simulink model "controller_class"  (R2024a)
settings: Solver=ode45  StartTime=0.0  StopTime=10  RelTol=1e-3
undefined symbols (not defined in the file or in its folder): Bi, BL, Bm_r, Bo, cmd, dis, f_t, J_r, Ji, Jo, K1_B, K1_B_H2, K2_B, K2_B_H2, K_A, K_A_H2, K_C, K_C_H2, KD_H2, Kd_w, Ke_r, Ki_d, KI_H2, Ki_i, Ki_w, KJB, KP_H2, Kp_i, Kp_w, Ks, Kt_r, L_r, R0, R_r, Ri, Ro, t_t, Vdc, Vp
libraries: simulink x2, fuzblock x1
settings Model: Creator=yanqi  LastModifiedBy=yanqi

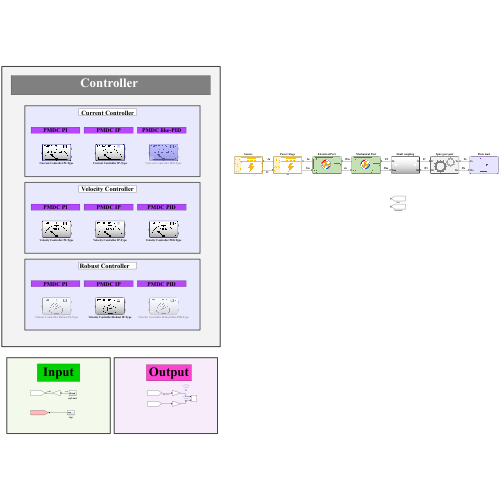
[thumbnail: Simulink's stored preview of the top-level diagram]
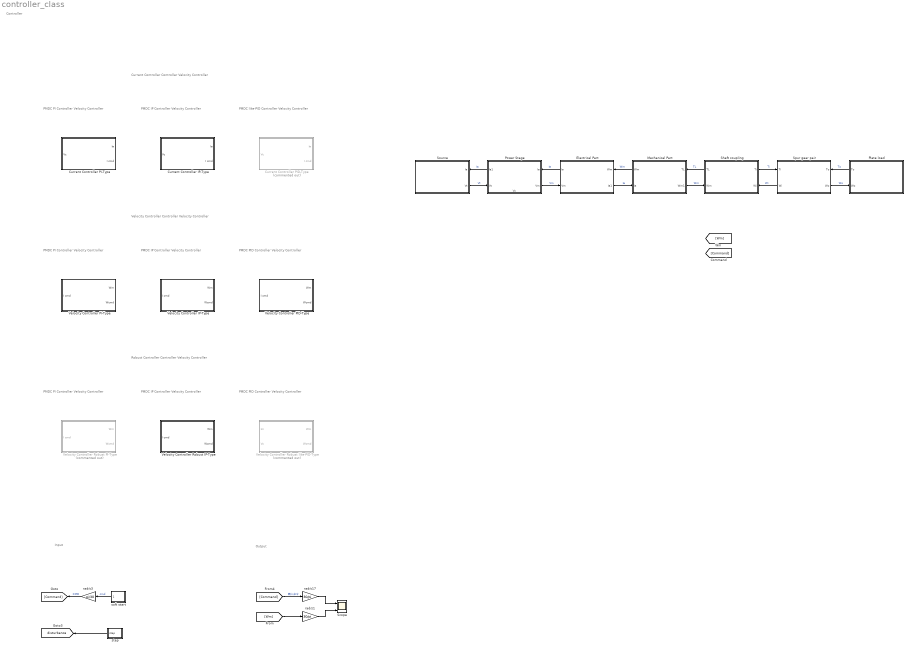
== system controller_class ==
  note: Current Controller Controller Velocity Controller
  note: PMDC IP Controller Velocity Controller
  note: PMDC like-PID Controller Velocity Controller
  note: PMDC PI Controller Velocity Controller
  note: Velocity Controller Controller Velocity Controller
  note: PMDC IP Controller Velocity Controller
  note: PMDC PID Controller Velocity Controller
  note: PMDC PI Controller Velocity Controller
  note: Robust Controller Controller Velocity Controller
  note: PMDC IP Controller Velocity Controller
  note: PMDC PID Controller Velocity Controller
  note: PMDC PI Controller Velocity Controller
  note: Controller
  note: Output
  note: Input
  Current Controller IP-Type : Subsystem  InitFcn=""
      mask Display: image("C:\Users\yanqi\Dropbox\強健控制\強健控制器設計\強健控制程式工具\TWO Port 模擬檔\可視化圖片\控制器\PMDC_Current_IP.png");
  Current Controller PI-Type : Subsystem  InitFcn=""
      mask Display: image("C:\Users\yanqi\Dropbox\強健控制\強健控制器設計\強健控制程式工具\TWO Port 模擬檔\可視化圖片\控制器\PMDC_Current_PI.png");
  Current Controller PID-Type : Subsystem  Commented=on  InitFcn=""
      mask Display: image("C:\Users\yanqi\Dropbox\強健控制\強健控制器設計\強健控制程式工具\TWO Port 模擬檔\可視化圖片\控制器\PMDC_Current_PID.png");
  Electrical Part : Subsystem
      settings: PortSchema="{\"entries\":[{\"content\":{\"sides\":[{\"content\":{\"connectorIds\":[\"Out2\",\"In1\"]},\"type\":\"ConnectorPlacement.EquallySpacedRectSide\",\"uuid\":\"f8a1ffa4-7450-4f3a-a88f-322599fa6d56\"},{\"content\":{\"connectorIds\":[\"In2\",\"Out1\"],\"side\":\"RIGHT\"},\"type\":\"ConnectorPlacement.EquallySpacedRectSide\",\"uuid\":\"f89fbec4-8dee-4bae-8289-3af4287f7f86\"},{\"content\":{\"side\":\"TOP\"},\"type\":\"ConnectorPlacement.EquallySpacedRectSide\",\"uuid\":\"83195871-21ad-4509-9495-08e0be9a8292\"}]},\"type\":\"ConnectorPlacement.EquallySpacedConnector\",\"uuid\":\"f8e5f4c3-4a70-47c9-aad6-1e160c7a2ed2\"}],\"packageUris\":[\"http://schema.mathworks.com/mf0/Connector/R2020b\"],\"version\":\"1.0\"}"
      mask Display: image('PMDC.png');
  Mechanical Part : Subsystem
      settings: PortSchema="{\"entries\":[{\"content\":{\"sides\":[{\"content\":{\"connectorIds\":[\"Out2\",\"In1\"]},\"type\":\"ConnectorPlacement.EquallySpacedRectSide\",\"uuid\":\"f8a1ffa4-7450-4f3a-a88f-322599fa6d56\"},{\"content\":{\"connectorIds\":[\"In2\",\"Out1\"],\"side\":\"RIGHT\"},\"type\":\"ConnectorPlacement.EquallySpacedRectSide\",\"uuid\":\"f89fbec4-8dee-4bae-8289-3af4287f7f86\"},{\"content\":{\"side\":\"TOP\"},\"type\":\"ConnectorPlacement.EquallySpacedRectSide\",\"uuid\":\"83195871-21ad-4509-9495-08e0be9a8292\"}]},\"type\":\"ConnectorPlacement.EquallySpacedConnector\",\"uuid\":\"f8e5f4c3-4a70-47c9-aad6-1e160c7a2ed2\"}],\"packageUris\":[\"http://schema.mathworks.com/mf0/Connector/R2020b\"],\"version\":\"1.0\"}"
      mask Display: image('PMDC.png');
  Plate load : Subsystem
      settings: PortSchema="{\"entries\":[{\"content\":{\"sides\":[{\"content\":{},\"type\":\"ConnectorPlacement.EquallySpacedRectSide\",\"uuid\":\"d42fc156-06c9-4c30-b734-ba7c649bcd6c\"},{\"content\":{\"side\":\"RIGHT\"},\"type\":\"ConnectorPlacement.EquallySpacedRectSide\",\"uuid\":\"e3421591-54ab-4525-97e2-f729a89143d8\"},{\"content\":{\"connectorIds\":[\"Out1\",\"In1\"],\"side\":\"TOP\"},\"type\":\"ConnectorPlacement.EquallySpacedRectSide\",\"uuid\":\"958f7cdf-8dcf-4bff-be32-b737eb42e197\"}]},\"type\":\"ConnectorPlacement.EquallySpacedConnector\",\"uuid\":\"ee7151ba-f83a-4c95-85b6-9993354922b3\"}],\"packageUris\":[\"http://schema.mathworks.com/mf0/Connector/R2020b\"],\"version\":\"1.0\"}"
      mask Display: image('LOAD.png');
  Power Stage : Subsystem
      settings: PortSchema="{\"entries\":[{\"content\":{\"sides\":[{\"content\":{\"connectorIds\":[\"Out2\",\"In1\"]},\"type\":\"ConnectorPlacement.EquallySpacedRectSide\",\"uuid\":\"58508ce2-1894-42d8-835a-89d3025a2a64\"},{\"content\":{\"connectorIds\":[\"In3\",\"Out1\"],\"side\":\"RIGHT\"},\"type\":\"ConnectorPlacement.EquallySpacedRectSide\",\"uuid\":\"6994be33-a1a7-4027-bab1-df4ce47b873a\"},{\"content\":{\"side\":\"TOP\"},\"type\":\"ConnectorPlacement.EquallySpacedRectSide\",\"uuid\":\"2ad4f745-7ac4-4e1a-9a98-a432c01e08ff\"},{\"content\":{\"connectorIds\":[\"In2\"],\"side\":\"BOTTOM\"},\"type\":\"ConnectorPlacement.EquallySpacedRectSide\",\"uuid\":\"1b30d730-4089-4eab-8923-76d29eb9f10c\"}]},\"type\":\"ConnectorPlacement.EquallySpacedConnector\",\"uuid\":\"b52e3181-20dc-4fdc-95a1-9a3597bd758e\"}],\"packageUris\":[\"http://schema.mathworks.com/mf0/Connector/R2020b\"],\"version\":\"1.0\"}"
      mask Display: image('DC Power.png');
  Scope : Scope  NumInputPorts=2
  Shaft coupling : Subsystem
      settings: PortSchema="{\"entries\":[{\"content\":{\"sides\":[{\"content\":{\"connectorIds\":[\"Out2\",\"In1\"]},\"type\":\"ConnectorPlacement.EquallySpacedRectSide\",\"uuid\":\"01ede124-f7d4-4ffa-a713-cf07b9ad0f27\"},{\"content\":{\"connectorIds\":[\"Out1\",\"In2\"],\"side\":\"RIGHT\"},\"type\":\"ConnectorPlacement.EquallySpacedRectSide\",\"uuid\":\"f66caf2a-ca8f-4ebf-97ad-d73b5315af29\"},{\"content\":{\"side\":\"TOP\"},\"type\":\"ConnectorPlacement.EquallySpacedRectSide\",\"uuid\":\"58e7144f-6e7e-4352-98b7-aac542d17719\"}]},\"type\":\"ConnectorPlacement.EquallySpacedConnector\",\"uuid\":\"1e1b0c9a-4571-49a4-a41d-a8591e57bca4\"}],\"packageUris\":[\"http://schema.mathworks.com/mf0/Connector/R2020b\"],\"version\":\"1.0\"}"
      mask Display: image('Rigid Coupling.png');
  Source : Subsystem
      settings: PortSchema="{\"entries\":[{\"content\":{\"sides\":[{\"content\":{},\"type\":\"ConnectorPlacement.EquallySpacedRectSide\",\"uuid\":\"717e91a0-288b-4ba5-84da-f262c24688bc\"},{\"content\":{\"connectorIds\":[\"In1\",\"Out1\"],\"side\":\"RIGHT\"},\"type\":\"ConnectorPlacement.EquallySpacedRectSide\",\"uuid\":\"569ee505-38fb-400b-9e45-0fafedafb0f3\"},{\"content\":{\"side\":\"TOP\"},\"type\":\"ConnectorPlacement.EquallySpacedRectSide\",\"uuid\":\"44407c3d-239d-4fc9-b2d2-10ddbad2f525\"}]},\"type\":\"ConnectorPlacement.EquallySpacedConnector\",\"uuid\":\"e894aa65-7991-48d5-91da-50bab94327d3\"}],\"packageUris\":[\"http://schema.mathworks.com/mf0/Connector/R2020b\"],\"version\":\"1.0\"}"
      mask Display: image('DC Power.png');
  Spur gear pair : Subsystem
      settings: PortSchema="{\"entries\":[{\"content\":{\"sides\":[{\"content\":{\"connectorIds\":[\"In1\",\"Out2\"]},\"type\":\"ConnectorPlacement.EquallySpacedRectSide\",\"uuid\":\"9ad50964-c829-49ed-8028-dcb862de1bdd\"},{\"content\":{\"connectorIds\":[\"In2\",\"Out1\"],\"side\":\"RIGHT\"},\"type\":\"ConnectorPlacement.EquallySpacedRectSide\",\"uuid\":\"a1a8b250-47a3-4252-871c-028bd872c8ce\"},{\"content\":{\"side\":\"TOP\"},\"type\":\"ConnectorPlacement.EquallySpacedRectSide\",\"uuid\":\"bcffd697-c189-4993-a911-6095dd8b92d6\"}]},\"type\":\"ConnectorPlacement.EquallySpacedConnector\",\"uuid\":\"be779869-a0ea-4cde-9a54-80cee426721f\"}],\"packageUris\":[\"http://schema.mathworks.com/mf0/Connector/R2020b\"],\"version\":\"1.0\"}"
      mask Display: image('Gear.png');
  Velocity Controller IP-Type : Subsystem  InitFcn=""
      mask Display: image("C:\Users\yanqi\Dropbox\強健控制\強健控制器設計\強健控制程式工具\TWO Port 模擬檔\可視化圖片\控制器\PMDC_Spped_IP.png");
  Velocity Controller PI-Type : Subsystem  InitFcn=""
      mask Display: image("C:\Users\yanqi\Dropbox\強健控制\強健控制器設計\強健控制程式工具\TWO Port 模擬檔\可視化圖片\控制器\PMDC_Spped_PI.png");
  Velocity Controller PID-Type : Subsystem  InitFcn=""
      mask Display: image("C:\Users\yanqi\Dropbox\強健控制\強健控制器設計\強健控制程式工具\TWO Port 模擬檔\可視化圖片\控制器\PMDC_Spped_PID.png");
  Velocity Controller Robust IP-Type : Subsystem  InitFcn=""
      mask Display: image("C:\Users\yanqi\Dropbox\強健控制\強健控制器設計\強健控制程式工具\TWO Port 模擬檔\可視化圖片\控制器\PMDC_Robust_IP.png");
  Velocity Controller Robust PI-Type : Subsystem  Commented=on  InitFcn=|
      | % P Matrix
      | H2_P = [-0.0953	0	0	1.9459	363.9515
      |         -1.0000	0	0.3410	-0.0021	0
      |         0	999.9800	0	0	0
      |         -0.2155	0	0	0	0
      |         0	0	0	0	0.0026
      |         0	1.0000	0.0011	0	0
      |         1.0000	0	0	0.0021	0];
      | 
      | %% H2 tool
      | [H2_A_T,H2_B_T,H2_C_T,H2_D_T,H2_A_K,H2_B_K,H2_C_K,H2_D_K,Norm] = H2_DF(H2_P,2,2,1,3,2);
      | 
      | % velocity controller
      | K_A_H2  = H2_A_K;
      | K1_B_H2 = H2_B_K(1:2,1);
      | K2_B_H2 = H2_B_K(1:2,2);
      | K_C_H2  = H2_C_K;
      mask Display: image("C:\Users\yanqi\Dropbox\強健控制\強健控制器設計\強健控制程式工具\TWO Port 模擬檔\可視化圖片\控制器\PMDC_Robust_PI.png");
  Velocity Controller Robust like-PID-Type : Subsystem  Commented=on  InitFcn=|
      | % P Matrix
      | H2_P = [-0.0953	0	0	1.9459	363.9515
      |         -1.0000	0	0.3410	-0.0021	0
      |         0	999.9800	0	0	0
      |         -0.2155	0	0	0	0
      |         0	0	0	0	0.0026
      |         0	1.0000	0.0011	0	0
      |         1.0000	0	0	0.0021	0];
      | 
      | %% H2 tool
      | [H2_A_T,H2_B_T,H2_C_T,H2_D_T,H2_A_K,H2_B_K,H2_C_K,H2_D_K,Norm] = H2_DF(H2_P,2,2,1,3,2);
      | 
      | % velocity controller
      | K_A_H2  = H2_A_K;
      | K1_B_H2 = H2_B_K(1:2,1);
      | K2_B_H2 = H2_B_K(1:2,2);
      | K_C_H2  = H2_C_K;
      settings: PortSchema="{\"entries\":[{\"content\":{\"sides\":[{\"content\":{\"connectorIds\":[\"In1\",\"In2\"]},\"type\":\"ConnectorPlacement.EquallySpacedRectSide\",\"uuid\":\"67442645-cd32-4145-b143-2bfd4b8863c1\"},{\"content\":{\"connectorIds\":[\"In3\",\"Out1\"],\"side\":\"RIGHT\"},\"type\":\"ConnectorPlacement.EquallySpacedRectSide\",\"uuid\":\"525717ef-81e8-4055-8109-230bda9ce61c\"},{\"content\":{\"side\":\"TOP\"},\"type\":\"ConnectorPlacement.EquallySpacedRectSide\",\"uuid\":\"18f89565-0718-45fc-8263-cc7fc51687c0\"}]},\"type\":\"ConnectorPlacement.EquallySpacedConnector\",\"uuid\":\"5a159387-e0fa-4e2f-b611-20c995e77047\"}],\"packageUris\":[\"http://schema.mathworks.com/mf0/Connector/R2020b\"],\"version\":\"1.0\"}"
      mask Display: image("C:\Users\yanqi\Dropbox\強健控制\強健控制器設計\強健控制程式工具\TWO Port 模擬檔\可視化圖片\控制器\PMDC_Robust_like-PID.png");
  rad/s1 : Gain  Gain=30/pi
  rad/s17 : Gain  Gain=30/pi
  rad/s3 : Gain  Gain=pi/30
  soft start : Subsystem
  step : Subsystem
  tag scope: disturbance=global
  wires:
  Shaft coupling/2(TL) -> Mechanical Part/2(TL)  "TL"
  Mechanical Part/1(Wm1) -> Shaft coupling/1(Wm)  "Wm"
  Source/1(Vt) -> Power Stage/1(Vt)  "Vt"
  Electrical Part/1(Ia1) -> Mechanical Part/1(Ia)  "Ia"
  Mechanical Part/2(Wm) -> Electrical Part/2(Wm)  "Wm"
  Power Stage/1(Vm) -> Electrical Part/1(Vm)  "Vm"
  Electrical Part/2(Ia) -> Power Stage/3(Ia)  "Ia"
  Power Stage/2(Ia1) -> Source/1(Ia)  "Ia"
  Shaft coupling/1(Ti) -> Spur gear pair/1(Ti)  "Ti"
  Spur gear pair/2(Wi) -> Shaft coupling/2(Wi)  "Wi"
  Spur gear pair/1(Wo) -> Plate load/1(Wo)  "Wo"
  Plate load/1(To) -> Spur gear pair/2(To)  "To"
  [Command] -> rad/s17/1  "轉入命令"
  rad/s17/1 -> Scope/1
  rad/s3/1 -> [Command]  "CMD"
  soft start/1(Wcmd) -> rad/s3/1  "cmd"
  rad/s1/1 -> Scope/2
  [Wm] -> rad/s1/1
  step/1(step) -> [disturbance]

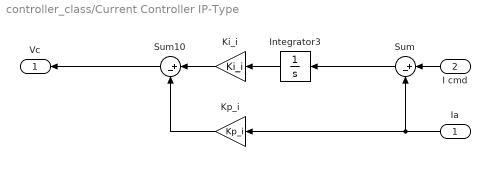
== system controller_class/Current Controller IP-Type ==
  Ia : Inport
  I cmd : Inport  Port=2
  Integrator3 : Integrator
  Ki_i : Gain  Gain=Ki_i
  Kp_i : Gain  Gain=Kp_i
  Sum : Sum  Inputs=|+-
  Sum10 : Sum  Inputs=|+-
  Vc : Outport
  wires:
  Integrator3/1 -> Ki_i/1
  Ki_i/1 -> Sum10/1
  Sum/1 -> Integrator3/1
  Sum10/1 -> Vc/1
  Ia/1 -> Sum/2, Kp_i/1
  I cmd/1 -> Sum/1
  Kp_i/1 -> Sum10/2

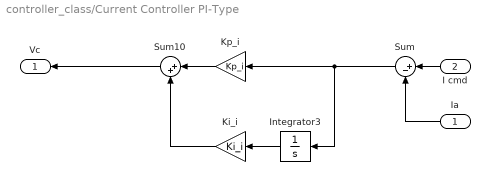
== system controller_class/Current Controller PI-Type ==
  Ia : Inport
  I cmd : Inport  Port=2
  Integrator3 : Integrator
  Ki_i : Gain  Gain=Ki_i
  Kp_i : Gain  Gain=Kp_i
  Sum : Sum  Inputs=|+-
  Sum10 : Sum  Inputs=|++
  Vc : Outport
  wires:
  I cmd/1 -> Sum/1
  Ia/1 -> Sum/2
  Sum10/1 -> Vc/1
  Sum/1 -> Integrator3/1, Kp_i/1
  Kp_i/1 -> Sum10/1
  Ki_i/1 -> Sum10/2
  Integrator3/1 -> Ki_i/1

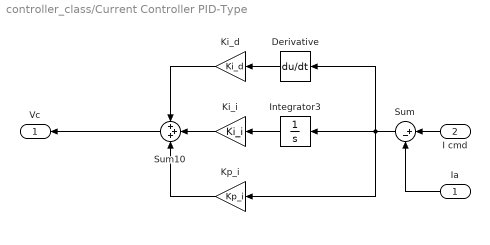
== system controller_class/Current Controller PID-Type ==
  Ia : Inport
  I cmd : Inport  Port=2
  Derivative : Derivative
  Integrator3 : Integrator
  Ki_d : Gain  Gain=Ki_d
  Ki_i : Gain  Gain=Ki_i
  Kp_i : Gain  Gain=Kp_i
  Sum : Sum  Inputs=|+-
  Sum10 : Sum  Inputs=+++
  Vc : Outport
  wires:
  I cmd/1 -> Sum/1
  Ia/1 -> Sum/2
  Sum10/1 -> Vc/1
  Sum/1 -> Derivative/1, Kp_i/1, Integrator3/1
  Integrator3/1 -> Ki_i/1
  Derivative/1 -> Ki_d/1
  Ki_i/1 -> Sum10/2
  Kp_i/1 -> Sum10/3
  Ki_d/1 -> Sum10/1

== system controller_class/Electrical Part ==
  Vm : Inport
  Wm : Inport  Port=2
  Sum18 : Sum  Inputs=|+-
  Transfer Fcn5 : TransferFcn  Denominator=[L_r R_r]
  反電動常數(V‧s/rad)2 : Gain  Gain=Ke_r
  Ia1 : Outport
  Ia : Outport  Port=2
  wires:
  Sum18/1 -> Transfer Fcn5/1
  反電動常數(V‧s/rad)2/1 -> Sum18/2  "V"
  Transfer Fcn5/1 -> Ia1/1, Ia/1
  Vm/1 -> Sum18/1
  Wm/1 -> 反電動常數(V‧s/rad)2/1

== system controller_class/Mechanical Part ==
  Ia : Inport
  TL : Inport  Port=2
  Sum19 : Sum  Inputs=-+|
  Transfer Fcn6 : TransferFcn  Denominator=[J_r Bm_r]
  扭矩常數(N．m/A)2 : Gain  Gain=Kt_r
  Wm1 : Outport
  Wm : Outport  Port=2
  wires:
  Transfer Fcn6/1 -> Wm1/1, Wm/1  "Wm"
  扭矩常數(N．m/A)2/1 -> Sum19/2  "Tem"
  Sum19/1 -> Transfer Fcn6/1
  TL/1 -> Sum19/1
  Ia/1 -> 扭矩常數(N．m/A)2/1

== system controller_class/Plate load ==
  Wo : Inport
  Gain : Gain  Gain=BL
  To : Outport
  wires:
  Wo/1 -> Gain/1
  Gain/1 -> To/1

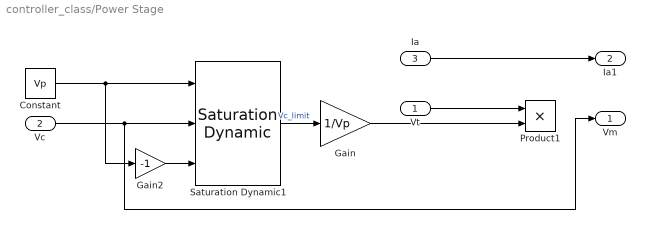
== system controller_class/Power Stage ==
  Vt : Inport
  Vc : Inport  Port=2
  Ia : Inport  Port=3
  Constant : Constant  Value=Vp
  Gain : Gain  Gain=1/Vp
  Gain2 : Gain  Gain=-1
  Product1 : Product
  Saturation Dynamic1 : simulink/Discontinuities/Saturation Dynamic  OutMin=[]  OutMax=[]  OutDataTypeStr=Inherit: Same as second input  OutDataType=fixdt(1, 16)  OutScaling=2^-10  DoSatur=off
  Vm : Outport
  Ia1 : Outport  Port=2
  wires:
  Ia/1 -> Ia1/1
  Gain2/1 -> Saturation Dynamic1/3
  Vc/1 -> Vm/1, Saturation Dynamic1/2
  Saturation Dynamic1/1 -> Gain/1  "Vc_limit"
  Constant/1 -> Saturation Dynamic1/1, Gain2/1
  Gain/1 -> Product1/2
  Vt/1 -> Product1/1

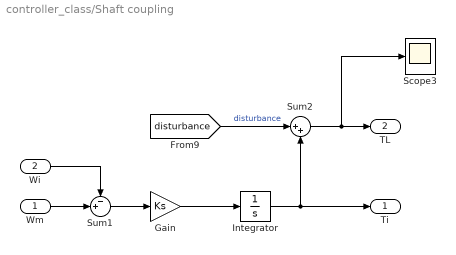
== system controller_class/Shaft coupling ==
  Wm : Inport
  Wi : Inport  Port=2
  Gain : Gain  Gain=Ks
  Integrator : Integrator
  Scope3 : Scope
  Sum1 : Sum  Inputs=-+|
  Sum2 : Sum  Inputs=|++
  Ti : Outport
  TL : Outport  Port=2
  wires:
  [disturbance] -> Sum2/1  "disturbance"
  Integrator/1 -> Ti/1, Sum2/2
  Sum2/1 -> TL/1, Scope3/1
  Sum1/1 -> Gain/1
  Gain/1 -> Integrator/1
  Wm/1 -> Sum1/2
  Wi/1 -> Sum1/1

== system controller_class/Source ==
  Ia : Inport
  Gain2 : Gain  Gain=R0
  Sum8 : Sum  Inputs=-+|
  Vin : Constant  Value=Vdc
  Vt : Outport
  wires:
  Ia/1 -> Gain2/1
  Vin/1 -> Sum8/2
  Sum8/1 -> Vt/1  "Vt"
  Gain2/1 -> Sum8/1

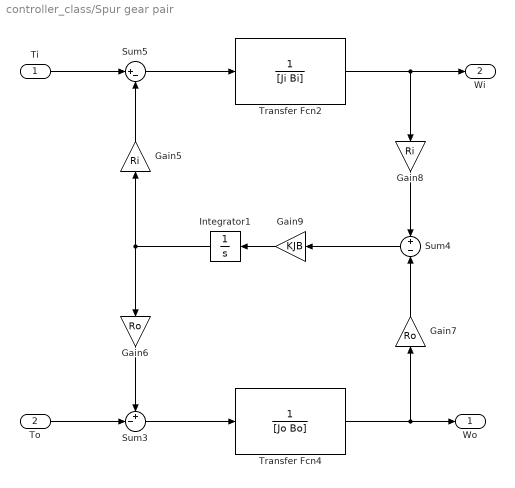
== system controller_class/Spur gear pair ==
  Ti : Inport
  To : Inport  Port=2
  Gain5 : Gain  Gain=Ri
  Gain6 : Gain  Gain=Ro
  Gain7 : Gain  Gain=Ro
  Gain8 : Gain  Gain=Ri
  Gain9 : Gain  Gain=KJB
  Integrator1 : Integrator
  Sum3 : Sum  Inputs=+-|
  Sum4 : Sum  Inputs=+|-
  Sum5 : Sum  Inputs=|+-
  Transfer Fcn2 : TransferFcn  Denominator=[Ji Bi]
  Transfer Fcn4 : TransferFcn  Denominator=[Jo Bo]
  Wo : Outport
  Wi : Outport  Port=2
  wires:
  Sum5/1 -> Transfer Fcn2/1
  To/1 -> Sum3/2
  Gain8/1 -> Sum4/1
  Sum3/1 -> Transfer Fcn4/1
  Gain6/1 -> Sum3/1
  Integrator1/1 -> Gain5/1, Gain6/1
  Ti/1 -> Sum5/1
  Transfer Fcn2/1 -> Gain8/1, Wi/1
  Gain9/1 -> Integrator1/1
  Gain7/1 -> Sum4/2
  Transfer Fcn4/1 -> Gain7/1, Wo/1
  Gain5/1 -> Sum5/2
  Sum4/1 -> Gain9/1

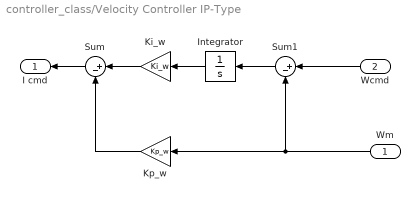
== system controller_class/Velocity Controller IP-Type ==
  Wm : Inport
  Wcmd : Inport  Port=2
  Integrator : Integrator
  Ki_w : Gain  Gain=Ki_w
  Kp_w : Gain  Gain=Kp_w
  Sum : Sum  Inputs=|+-
  Sum1 : Sum  Inputs=|+-
  I cmd : Outport
  wires:
  Sum/1 -> I cmd/1
  Wcmd/1 -> Sum1/1
  Wm/1 -> Kp_w/1, Sum1/2
  Sum1/1 -> Integrator/1
  Kp_w/1 -> Sum/2
  Ki_w/1 -> Sum/1
  Integrator/1 -> Ki_w/1

== system controller_class/Velocity Controller PI-Type ==
  Wm : Inport
  Wcmd : Inport  Port=2
  Integrator : Integrator
  Ki_w : Gain  Gain=Ki_w
  Kp_w : Gain  Gain=Kp_w
  Sum : Sum  Inputs=|++
  Sum1 : Sum  Inputs=|+-
  I cmd : Outport
  wires:
  Integrator/1 -> Ki_w/1
  Ki_w/1 -> Sum/1
  Kp_w/1 -> Sum/2
  Sum1/1 -> Kp_w/1, Integrator/1
  Wm/1 -> Sum1/2
  Wcmd/1 -> Sum1/1
  Sum/1 -> I cmd/1

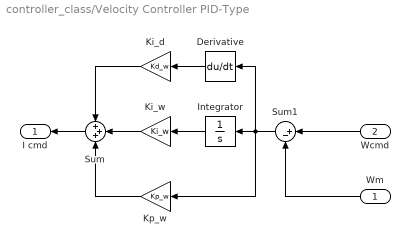
== system controller_class/Velocity Controller PID-Type ==
  Wm : Inport
  Wcmd : Inport  Port=2
  Derivative : Derivative
  Integrator : Integrator
  Ki_d : Gain  Gain=Kd_w
  Ki_w : Gain  Gain=Ki_w
  Kp_w : Gain  Gain=Kp_w
  Sum : Sum  Inputs=+++
  Sum1 : Sum  Inputs=|+-
  I cmd : Outport
  wires:
  Integrator/1 -> Ki_w/1
  Wcmd/1 -> Sum1/1
  Sum/1 -> I cmd/1
  Wm/1 -> Sum1/2
  Derivative/1 -> Ki_d/1
  Sum1/1 -> Derivative/1, Kp_w/1, Integrator/1
  Ki_d/1 -> Sum/1
  Kp_w/1 -> Sum/3
  Ki_w/1 -> Sum/2

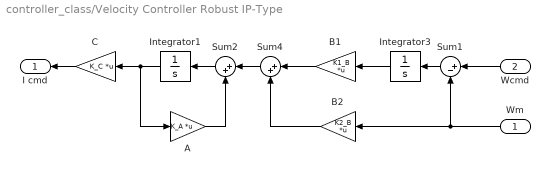
== system controller_class/Velocity Controller Robust IP-Type ==
  Wm : Inport
  Wcmd : Inport  Port=2
  A : Gain  Gain=K_A  Multiplication=Matrix(K*u)
  B1 : Gain  Gain=K1_B  Multiplication=Matrix(K*u)
  B2 : Gain  Gain=K2_B  Multiplication=Matrix(K*u)
  C : Gain  Gain=K_C  Multiplication=Matrix(K*u)
  Integrator1 : Integrator
  Integrator3 : Integrator
  Sum1 : Sum  Inputs=|+-
  Sum2 : Sum  Inputs=|++
  Sum4 : Sum  Inputs=|++
  I cmd : Outport
  wires:
  C/1 -> I cmd/1
  Wcmd/1 -> Sum1/1
  Integrator3/1 -> B1/1
  Sum1/1 -> Integrator3/1
  B1/1 -> Sum4/1
  A/1 -> Sum2/2
  B2/1 -> Sum4/2
  Sum2/1 -> Integrator1/1
  Sum4/1 -> Sum2/1
  Integrator1/1 -> A/1, C/1
  Wm/1 -> B2/1, Sum1/2

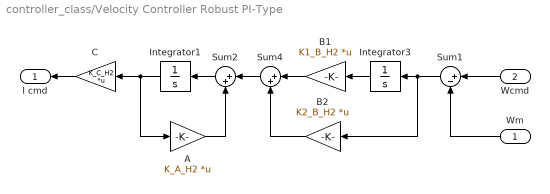
== system controller_class/Velocity Controller Robust PI-Type ==
  Wm : Inport
  Wcmd : Inport  Port=2
  A : Gain  Gain=K_A_H2  Multiplication=Matrix(K*u)
  B1 : Gain  Gain=K1_B_H2  Multiplication=Matrix(K*u)
  B2 : Gain  Gain=K2_B_H2  Multiplication=Matrix(K*u)
  C : Gain  Gain=K_C_H2  Multiplication=Matrix(K*u)
  Integrator1 : Integrator
  Integrator3 : Integrator
  Sum1 : Sum  Inputs=|+-
  Sum2 : Sum  Inputs=|++
  Sum4 : Sum  Inputs=|++
  I cmd : Outport
  wires:
  Wm/1 -> Sum1/2
  Integrator1/1 -> C/1, A/1
  Sum4/1 -> Sum2/1
  Sum2/1 -> Integrator1/1
  B2/1 -> Sum4/2
  A/1 -> Sum2/2
  B1/1 -> Sum4/1
  Sum1/1 -> B2/1, Integrator3/1
  Integrator3/1 -> B1/1
  Wcmd/1 -> Sum1/1
  C/1 -> I cmd/1

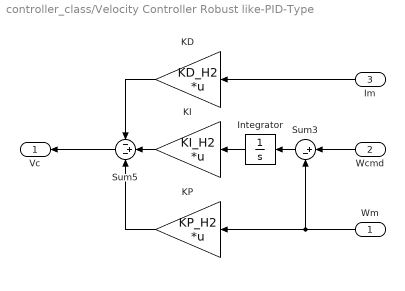
== system controller_class/Velocity Controller Robust like-PID-Type ==
  Wm : Inport
  Wcmd : Inport  Port=2
  Im : Inport  Port=3
  Integrator : Integrator
  KD : Gain  Gain=KD_H2  Multiplication=Matrix(K*u)
  KI : Gain  Gain=KI_H2  Multiplication=Matrix(K*u)
  KP : Gain  Gain=KP_H2  Multiplication=Matrix(K*u)
  Sum3 : Sum  Inputs=|+-
  Sum5 : Sum  Inputs=-+-
  Vc : Outport
  wires:
  Wm/1 -> KP/1, Sum3/2
  Im/1 -> KD/1
  KD/1 -> Sum5/1
  KI/1 -> Sum5/2
  Sum3/1 -> Integrator/1
  Wcmd/1 -> Sum3/1
  KP/1 -> Sum5/3
  Sum5/1 -> Vc/1
  Integrator/1 -> KI/1

== system controller_class/soft start ==
  Product : Product
  Ramp1 : simulink/Sources/Ramp  slope=1  start=0.1  InitialOutput=0
  S-shaped MF : fuzblock/Membership  Functions/S-shaped MF  a=0.3  b=3
  Step : Step  Time=0.1  After=cmd  SampleTime=0
  Wcmd : Outport
  wires:
  Ramp1/1 -> S-shaped MF/1
  S-shaped MF/1 -> Product/1
  Step/1 -> Product/2
  Product/1 -> Wcmd/1

== system controller_class/step ==
  Step : Step  Time=f_t  After=dis  SampleTime=0
  Step1 : Step  Time=t_t  After=dis  SampleTime=0
  Sum16 : Sum  Inputs=-+|
  step : Outport
  wires:
  Step/1 -> Sum16/2
  Step1/1 -> Sum16/1
  Sum16/1 -> step/1
